simulink model "SimulatedNetwork2"  (Simulink 8.2)
settings: Solver=FixedStepDiscrete  StartTime=0.0  StopTime=10  FixedStep=Ts  RelTol=1e-3
undefined symbols (not defined in the file or in its folder): P, sampPerFrame, seed
undefined symbols (not defined in the file): E1, E2, H1, H2, mu1, mu2, S1, S2
libraries: cstblocks x6, dspsrcs4 x2
settings Model: Creator=Developer  LastModifiedBy=iahncajigas
settings HardwareCC: TargetBitPerLong=64  TargetBitPerPointer=64  TargetLongLongMode=on  TargetIntDivRoundTo=Zero  TargetEndianess=LittleEndian  TargetWordSize=64  TargetHWDeviceType=MATLAB Host  ProdEqTarget=off
settings RTWCC: ProcessScript=grt_make_rtw_hook  RTWCompilerOptimization=On

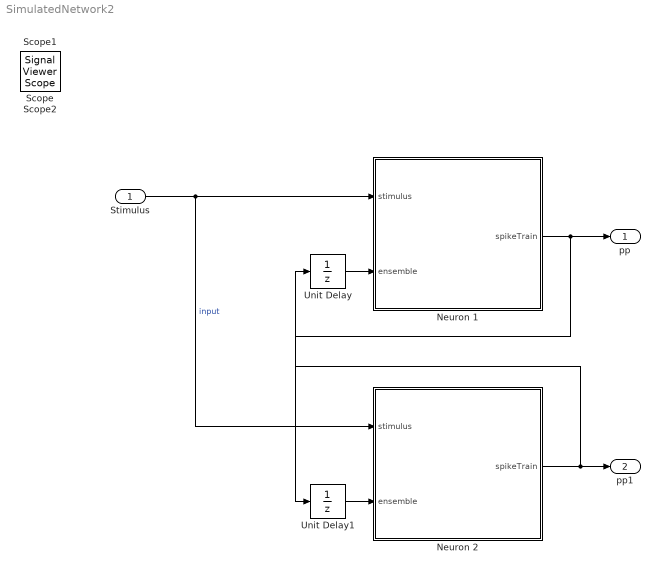
== system SimulatedNetwork2 ==
  Stimulus : Inport
  Neuron 1 : Subsystem  mask{H=H1, E=E1, S=S1, mu=mu1}
      mask prompts: H "History Filter"; E "Ensemble Filter"; S "Stimulus Filter"; mu "Baseline Firing Rate"
  Neuron 2 : Subsystem  mask{H=H2, E=E2, S=S2, mu=mu2}
      mask prompts: H "History Filter"; E "Ensemble Filter"; S "Stimulus Filter"; mu "Baseline Firing Rate"
  Unit Delay : UnitDelay  SampleTime=-1
  Unit Delay1 : UnitDelay  SampleTime=-1
  pp : Outport
  pp1 : Outport  Port=2
  Scope : SignalViewerScope  IOType=viewer  RefreshTime=0.035000
  Scope1 : SignalViewerScope  IOType=viewer  RefreshTime=0.035000
  Scope2 : SignalViewerScope  IOType=viewer  RefreshTime=0.035000
      settings: SaveName=ScopeData2
  wires:
  Stimulus/1 -> Neuron 1/1(stimulus), Neuron 2/1(stimulus)  "input"
  Neuron 1/1(spikeTrain) -> pp/1, Unit Delay1/1
  Neuron 2/1(spikeTrain) -> pp1/1, Unit Delay/1
  Unit Delay1/1 -> Neuron 2/2(ensemble)
  Unit Delay/1 -> Neuron 1/2(ensemble)

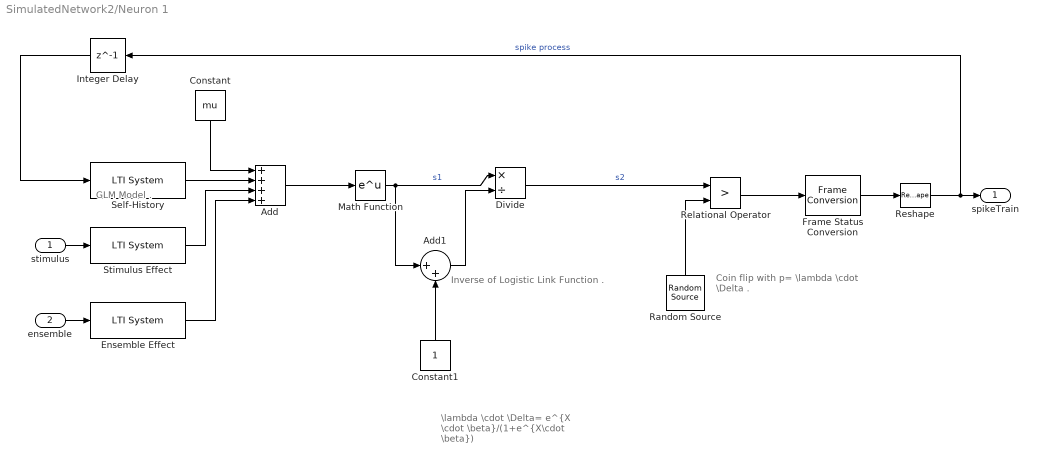
== system SimulatedNetwork2/Neuron 1 ==
  note: GLM Model
      |
      |
      |
      |
      |
      |
      |
      |
      |
      |
      |
      |
      |
      |
      |
      |
      |
      |
      | .
  note: Coin flip with
      | p= \lambda \cdot \Delta
      |
      |
      |
      |
      |
      |
      |
      |
      |
      |
      | .
  note: Inverse of Logistic Link Function
      |
      |
      |
      |
      |
      |
      |
      |
      |
      |
      | .
  note: \lambda \cdot \Delta= e^{X \cdot \beta}/(1+e^{X\cdot \beta})
  stimulus : Inport
  ensemble : Inport  Port=2
  Add : Sum  Inputs=++++
  Add1 : Sum  Inputs=|++
  Constant : Constant  Value=mu
  Constant1 : Constant
  Divide : Product  Inputs=*/
  Ensemble Effect : cstblocks/LTI System  sys=E  IC=[]
  Frame Status Conversion : FrameConversion  OutFrame=Sample-based
  Integer Delay : Delay  DelayLength=1
  Math Function : Math  SaturateOnIntegerOverflow=on
  Random Source : dspsrcs4/Random Source  SrcType=Uniform  NormMethod=Ziggurat  CltLength=12  MinVal=0  MaxVal=1  MeanVal=0  VarVal=1  RepMode=Not repeatable  rawSeed=seed  IsInherit=on  SampMode=Continuous  SampTime=Ts  SampFrame=dsp_sampFrame  DataType=Double  OutComplex=Real
  Relational Operator : RelationalOperator  Operator=>  OutDataTypeStr=float('double')  InputSameDT=on
  Reshape : Reshape  OutputDimensions=[sampPerFrame,max(length(P),length(seed))]
  Self-History : cstblocks/LTI System  sys=H  IC=[]
  Stimulus Effect : cstblocks/LTI System  sys=S  IC=[]
  spikeTrain : Outport
  wires:
  Constant/1 -> Add/1
  Self-History/1 -> Add/2
  Stimulus Effect/1 -> Add/3
  Add/1 -> Math Function/1
  Frame Status Conversion/1 -> Reshape/1
  Reshape/1 -> Integer Delay/1, spikeTrain/1  "spike process"
  Relational Operator/1 -> Frame Status Conversion/1
  Random Source/1 -> Relational Operator/2
  Integer Delay/1 -> Self-History/1
  Constant1/1 -> Add1/2
  Math Function/1 -> Add1/1, Divide/1  "s1"
  Add1/1 -> Divide/2
  Divide/1 -> Relational Operator/1  "s2"
  Ensemble Effect/1 -> Add/4
  stimulus/1 -> Stimulus Effect/1
  ensemble/1 -> Ensemble Effect/1

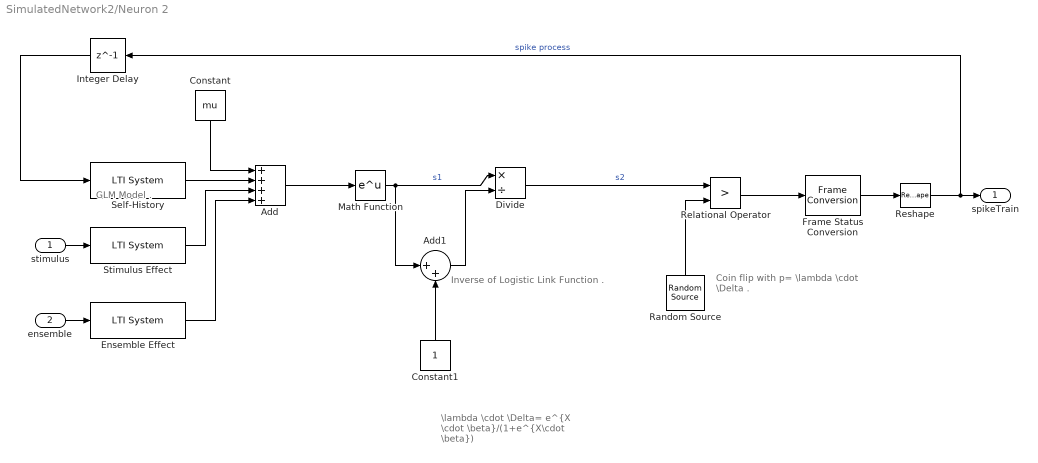
== system SimulatedNetwork2/Neuron 2 ==
  note: GLM Model
      |
      |
      |
      |
      |
      |
      |
      |
      |
      |
      |
      |
      |
      |
      |
      |
      |
      |
      | .
  note: Coin flip with
      | p= \lambda \cdot \Delta
      |
      |
      |
      |
      |
      |
      |
      |
      |
      |
      | .
  note: Inverse of Logistic Link Function
      |
      |
      |
      |
      |
      |
      |
      |
      |
      |
      | .
  note: \lambda \cdot \Delta= e^{X \cdot \beta}/(1+e^{X\cdot \beta})
  stimulus : Inport
  ensemble : Inport  Port=2
  Add : Sum  Inputs=++++
  Add1 : Sum  Inputs=|++
  Constant : Constant  Value=mu
  Constant1 : Constant
  Divide : Product  Inputs=*/
  Ensemble Effect : cstblocks/LTI System  sys=E  IC=[]
  Frame Status Conversion : FrameConversion  OutFrame=Sample-based
  Integer Delay : Delay  DelayLength=1
  Math Function : Math  SaturateOnIntegerOverflow=on
  Random Source : dspsrcs4/Random Source  SrcType=Uniform  NormMethod=Ziggurat  CltLength=12  MinVal=0  MaxVal=1  MeanVal=0  VarVal=1  RepMode=Not repeatable  rawSeed=seed  IsInherit=on  SampMode=Continuous  SampTime=Ts  SampFrame=dsp_sampFrame  DataType=Double  OutComplex=Real
  Relational Operator : RelationalOperator  Operator=>  OutDataTypeStr=float('double')  InputSameDT=on
  Reshape : Reshape  OutputDimensions=[sampPerFrame,max(length(P),length(seed))]
  Self-History : cstblocks/LTI System  sys=H  IC=[]
  Stimulus Effect : cstblocks/LTI System  sys=S  IC=[]
  spikeTrain : Outport
  wires:
  Constant/1 -> Add/1
  Self-History/1 -> Add/2
  Stimulus Effect/1 -> Add/3
  Add/1 -> Math Function/1
  Frame Status Conversion/1 -> Reshape/1
  Reshape/1 -> Integer Delay/1, spikeTrain/1  "spike process"
  Relational Operator/1 -> Frame Status Conversion/1
  Random Source/1 -> Relational Operator/2
  Integer Delay/1 -> Self-History/1
  Constant1/1 -> Add1/2
  Math Function/1 -> Add1/1, Divide/1  "s1"
  Add1/1 -> Divide/2
  Divide/1 -> Relational Operator/1  "s2"
  Ensemble Effect/1 -> Add/4
  stimulus/1 -> Stimulus Effect/1
  ensemble/1 -> Ensemble Effect/1
